simulink model "teste_motor_v10"  (R2025b)
settings: Solver=VariableStepAuto  StartTime=0.0  StopTime=10  RelTol=1e-3
undefined symbols (not defined in the file): fdesignblkfcn, gcbh, Kad, Kre
libraries: nesl_utility x26, fl_lib x25, simulink x19, dsparch4 x3, sdl_lib x2, simulink_extras x2, dspfdesign x1
(part 2 of 3)

== system teste_motor_v10/Motor de Sem Controle/Subsystem/Leituras/Janela ==
  In1 : Inport
  Aleatório : Subsystem
  Constant : Constant  Value=2
  Gain : Gain  Gain=1.5
  Janela : Subsystem
  Multiport Switch : MultiPortSwitch  SaturateOnIntegerOverflow=off  InputSameDT=off
  Product : Product
  Rotary Switch1 : CustomTuningWebBlock  LabelPosition=Hide  ShowInitialText=on  Configuration="{\"components\":[{\"name\":\"RotarySwitchComponent\",\"settings\":{\"arcAngle\":300,\"arcAngleOffset\":120,\"handle\":{\"size\":[150,150],\"src\":\"data:image\\/svg+xml;base64,PHN2ZyBpZD0iTGF5ZXJfMSIgZGF0YS1uYW1lPSJMYXllciAxIiB4bWxucz0iaHR0cDovL3d3dy53My5vcmcvMjAwMC9zdmciIHhtbG5zOnhsaW5rPSJodHRwOi8vd3d3LnczLm9yZy8xOTk5L3hsaW5rIiB2aWV3Qm94PSIwIDAgMTIxIDEyMSI+PGRlZnM+PHN0eWxlPi5jbHMtMXtmaWxsOnVybCgjbGluZWFyLWdyYWRpZW50KTt9LmNscy0yLC5jbHMtM3tmaWxsOiNkMWQxZDE7fS5jbHMtM3tzdHJva2U6I2I3YjdiNztzdHJva2UtbWl0ZXJsaW1pdDoxMDtzdHJva2Utd2lkdGg6MC4yNXB4O30uY2xzLTR7ZmlsbDojZjMwMDAwO30uY2xzLTV7ZmlsbDojZjIxNzY3O308L3N0eWxlPjxsaW5lYXJHcmFkaWVudCBpZD0ibGluZWFyLWdyYWRpZW50IiB4MT0iNjAuNSIgeTE9IjEyMC41IiB4Mj0iNjAuNSIgeTI9IjAuNSIgZ3JhZGllbnRVbml0cz0idXNlclNwYWNlT25Vc2UiPjxzdG9wIG9mZnNldD0iMCIgc3RvcC1jb2xvcj0iI2QxZDFkMSIvPjxzdG9wIG9mZnNldD0iMC4xIiBzdG9wLWNvbG9yPSIjY2VjZWNlIi8+PHN0b3Agb2Zmc2V0PSIwLjE5IiBzdG9wLWNvbG9yPSIjYzNjM2MzIi8+PHN0b3Agb2Zmc2V0PSIwLjI4IiBzdG9wLWNvbG9yPSIjYjFiMWIxIi8+PHN0b3Agb2Zmc2V0PSIwLjM2IiBzdG9wLWNvbG9yPSIjOTg5ODk4Ii8+PHN0b3Agb2Zmc2V0PSIwLjQ0IiBzdG9wLWNvbG9yPSIjNzg3ODc4Ii8+PHN0b3Agb2Zmc2V0PSIwLjQ2IiBzdG9wLWNvbG9yPSIjNmI2YjZiIi8+PHN0b3Agb2Zmc2V0PSIwLjU0IiBzdG9wLWNvbG9yPSIjNmI2YjZiIi8+PHN0b3Agb2Zmc2V0PSIwLjU2IiBzdG9wLWNvbG9yPSIjNzY3Njc2Ii8+PHN0b3Agb2Zmc2V0PSIwLjY0IiBzdG9wLWNvbG9yPSIjOTc5Nzk3Ii8+PHN0b3Agb2Zmc2V0PSIwLjcyIiBzdG9wLWNvbG9yPSIjYjBiMGIwIi8+PHN0b3Agb2Zmc2V0PSIwLjgxIiBzdG9wLWNvbG9yPSIjYzNjM2MzIi8+PHN0b3Agb2Zmc2V0PSIwLjkiIHN0b3AtY29sb3I9IiNjZGNkY2QiLz48c3RvcCBvZmZzZXQ9IjEiIHN0b3AtY29sb3I9IiNkMWQxZDEiLz48L2xpbmVhckdyYWRpZW50PjwvZGVmcz48Y2lyY2xlIGNsYXNzPSJjbHMtMSIgY3g9IjYwLjUiIGN5PSI2MC41IiByPSI2MCIvPjxwYXRoIGNsYXNzPSJjbHMtMiIgZD0iTTYwLjUsMUE1OS41LDU5LjUsMCwxLDEsMSw2MC41LDU5LjU3LDU5LjU3LDAsMCwxLDYwLjUsMW0wLTFBNjAuNSw2MC41LDAsMSwwLDEyMSw2MC41LDYwLjUsNjAuNSwwLDAsMCw2MC41LDBaIi8+PHJlY3QgY2xhc3M9ImNscy0zIiB4PSIwLjUiIHk9IjUxLjUiIHdpZHRoPSIxMjAiIGhlaWdodD0iMTgiIHJ4PSIzLjA0Ii8+PHJlY3QgY2xhc3M9ImNscy00IiB4PSI1Ljc1IiB5PSI1OC43NSIgd2lkdGg9IjE2IiBoZWlnaHQ9IjMiLz48cGF0aCBjbGFzcz0iY2xzLTUiIGQ9Ik0yMS4yNSw1OS4yNXYyaC0xNXYtMmgxNW0xLTFoLTE3djRoMTd2LTRaIi8+PC9zdmc+\"},\"handleOffset\":[0,0],\"handleOrientation\":180,\"handlePosition\":[0,0,1,1],\"handleSize\":{\"height\":0.5,\"width\":0.5},\"labelRadius\":0.36,\"position\":[0,0,1,1],\"states\":[{\"Label\":{\"color\":[0,0,0,1],\"icon\":{\"size\":[0,0],\"src\":[],\"srcOrientation\":\"Right\"},\"iconOffset\":0,\"iconPlacement\":\"left\",\"opacity\":1,\"position\":[0.35757211538461536,0.7603966346153846],\"show\":true,\"text\":{\"content\":\"Test\",\"font\":\"Helvetica\"}},\"Value\":1},{\"Label\":{\"color\":[0,0,0,1],\"icon\":{\"size\":[0,0],\"src\":[],\"srcOrientation\":\"Right\"},\"iconOffset\":0,\"iconPlacement\":\"left\",\"opacity\":1,\"position\":[0.09603365384615385,0.46033653846153844],\"show\":true,\"text\":{\"content\":\"Random\",\"font\":\"Helvetica\"}},\"Value\":2},{\"Label\":{\"color\":[0,0,0,1],\"icon\":{\"size\":[0,0],\"src\":[],\"srcOrientation\":\"Right\"},\"iconOffset\":0,\"iconPlacement\":\"left\",\"opacity\":1,\"position\":[0.36532451923076925,0.1180889423076923],\"show\":true,\"text\":{\"content\":\"Sequel\",\"font\":\"Helvetica\"}},\"Value\":3}],\"tickRadius\":0.32}},{\"name\":\"BackgroundImageComponent\",\"settings\":{\"image\":{\"size\":[155,150],\"src\":\"data:image\\/svg+xml;base64,PD94bWwgdmVyc2lvbj0iMS4wIiBlbmNvZGluZz0idXRmLTgiPz4NCjwhLS0gR2VuZXJhdG9yOiBBZG9iZSBJbGx1c3RyYXRvciAyNS4wLjAsIFNWRyBFeHBvcnQgUGx1Zy1JbiAuIFNWRyBWZXJzaW9uOiA2LjAwIEJ1aWxkIDApICAtLT4NCjxzdmcgdmVyc2lvbj0iMS4xIg0KCSBpZD0iTGF5ZXJfMl8xXyIgeG1sbnM6Y2M9Imh0dHA6Ly9jcmVhdGl2ZWNvbW1vbnMub3JnL25zIyIgeG1sbnM6ZGM9Imh0dHA6Ly9wdXJsLm9yZy9kYy9lbGVtZW50cy8xLjEvIiB4bWxuczppbmtzY2FwZT0iaHR0cDovL3d3dy5pbmtzY2FwZS5vcmcv ...(+4184 chars)\",\"srcOrientation\":\"Right\"},\"position\":[0,0,1,1],\"scaleMode\":\"0\"}},{\"name\":\"ForegroundImageComponent\",\"settings\":{\"image\":{\"size\":[0,0],\"src\":\"default\",\"srcOrientation\":[]},\"isForeground\":1,\"position\":[0,0,1,1],\"scaleMode\":\"0\"}}],\"derived\":{\"blockParameters\":{\"ForegroundColor\":[0.9882352941176471,0.9882352941176471,0.7725490196078432],\"SelectedStateIndex\":0,\"States\":[{\"Label\":{\"color\":[0,0,0,1],\"icon\":{\"size\":[0,0],\"src\":[],\"srcOrientation\":\"Right\"},\"iconOffset\":0,\"iconPlacement\":\"left\",\"opacity\":1,\"position\":[0.35757211538461536,0.7603966346153846],\"show\":true,\"text\":{\"content\":\"Test\",\"font\":\"Helvetica\"}},\"Value\":1},{\"Label\":{\"color\":[0,0,0,1],\"icon\":{\"size\":[0,0],\"src\":[],\"srcOrientation\":\"Right\"},\"iconOffset\":0,\"iconPlacement\":\"left\",\"opacity\":1,\"position\":[0.09603365384615385,0.46033653846153844],\"show\":true,\"text\":{\"content\":\"Random\",\"font\":\"Helvetica\"}},\"Value\":2},{\"Label\":{\"color\":[0,0,0,1],\"icon\":{\"size\":[0,0],\"src\":[],\"srcOrientation\":\"Right\"},\"iconOffset\":0,\"iconPlacement\":\"left\",\"opacity\":1,\"position\":[0.36532451923076925,0.1180889423076923],\"show\":true,\"text\":{\"content\":\"Sequel\",\"font\":\"Helvetica\"}},\"Value\":3}],\"StatesJSON\":[{\"Label\":\"Test\",\"Value\":1},{\"Label\":\"Random\",\"Value\":2},{\"Label\":\"Sequel\",\"Value\":3}],\"enumDataType\":\"\",\"fixedAspectRatio\":\"on\",\"useEnumDataType\":false}},\"settings\":{\"BindingType\":\"param\",\"backgroundColor\":[0,0,255,\"1\"],\"backgroundOffset\":1,\"fixedAspectRatio\":\"on\",\"image\":{\"size\":[150,150],\"src\":\"data:image\\/svg+xml;base64,PD94bWwgdmVyc2lvbj0iMS4wIiBlbmNvZGluZz0iVVRGLTgiIHN0YW5kYWxvbmU9Im5vIj8+CjwhLS0gR2VuZXJhdG9yOiBBZG9iZSBJbGx1c3RyYXRvciAxOS4yLjEsIFNWRyBFeHBvcnQgUGx1Zy1JbiAuIFNWRyBWZXJzaW9uOiA2LjAwIEJ1aWxkIDApICAtLT4KCjxzdmcKICAgeG1sbnM6ZGM9Imh0dHA6Ly9wdXJsLm9yZy9kYy9lbGVtZW50cy8xLjEvIgogICB4bWxuczpjYz0iaHR0cDovL2NyZWF0aXZlY29tbW9ucy5vcmcvbnMjIgogICB4bWxuczpyZGY9Imh0dHA6Ly93d3cudzMub3JnLzE5OTkvMDIvMjItcmRmLXN5bnRh ...(+9660 chars)\"},\"showBackgroundColor\":false,\"variant\":\"rotarySwitch\",\"version\":\"R2023a\"},\"type\":\"RotarySwitch\"}"
  Sequência : Subsystem
  Teste : Subsystem
  Out1 : Outport
  wires:
  In1/1 -> Janela/1(In1)
  Janela/1(Output) -> Product/2
  Product/1 -> Gain/1
  Gain/1 -> Out1/1
  Constant/1 -> Multiport Switch/1
  Teste/1(Out1) -> Multiport Switch/2
  Sequência/1(3) -> Multiport Switch/4
  Aleatório/1(2) -> Multiport Switch/3
  Multiport Switch/1 -> Product/1

== system teste_motor_v10/Motor de Sem Controle/Subsystem/Leituras/Knock ==
  In1 : Inport
  Abs1 : Abs  SaturateOnIntegerOverflow=off
  MATLAB Function : MATLAB Function  TreatAsAtomicUnit=on
  Product : Product  Inputs=3
  Transfer Fcn : TransferFcn  Denominator=[0.0002 1]
  Uniform Random Number : UniformRandomNumber  Minimum=1800  Maximum=2000  SampleTime=0.0001
  Waveform Generator : simulink/Sources/Waveform Generator  OutMin=[]  OutMax=[]  OutDataTypeStr=double  SelectedSignal=1  Signals=sin(1,80000,1)  BlockNames=MultiportSwitch_adaf1d14f166474  SampleTime=0.1
  Out1 : Outport
  wires:
  Waveform Generator/1 -> Abs1/1
  Transfer Fcn/1 -> Product/3
  Abs1/1 -> Product/2
  Product/1 -> Out1/1
  In1/1 -> Transfer Fcn/1
  MATLAB Function/1(knock_probabilidade) -> Product/1
  [rpm] -> MATLAB Function/1(rpm)
  [AFR] -> MATLAB Function/2(AFR)
  [sa] -> MATLAB Function/3(SA)

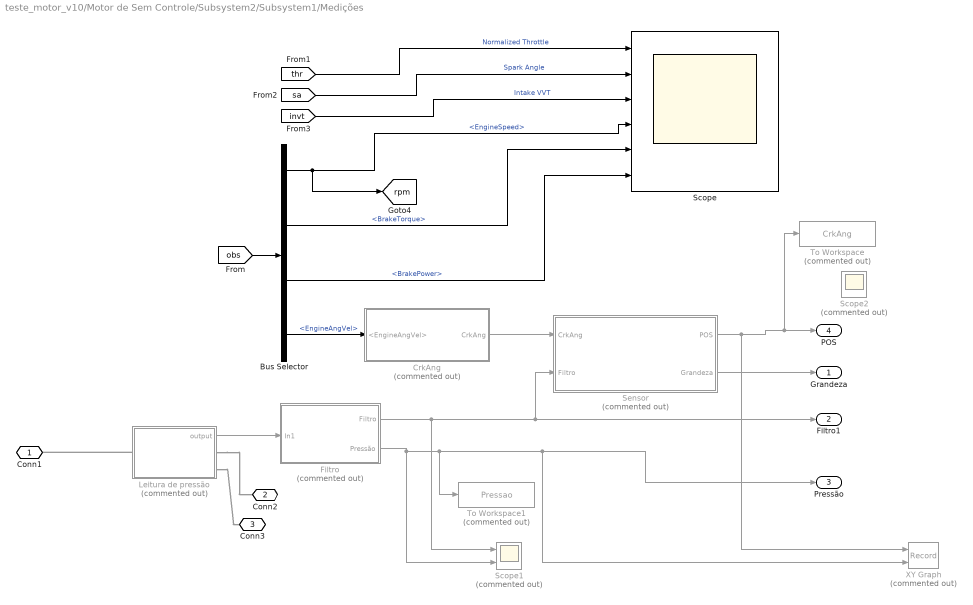
== system teste_motor_v10/Motor de Sem Controle/Subsystem2/Subsystem1/Medições ==
  Bus Selector : BusSelector  OutputSignals=EngineSpeed,BrakeTorque,BrakePower,EngineAngVel
  CrkAng : Subsystem  Commented=on
  Filtro : Subsystem  Commented=on
  Leitura de pressão : Subsystem  Commented=on
  Scope : Scope  NumInputPorts=6
      settings: ActiveDisplayYMinimum=0.1  ActiveDisplayYMaximum=1.1
  Scope1 : Scope  Commented=on  NumInputPorts=2
      settings: ActiveDisplayYMinimum=-2759.66095  ActiveDisplayYMaximum=3628.39198  DataLoggingVariableName=ScopeData3
  Scope2 : Scope  Commented=on
      settings: ActiveDisplayYMinimum=-46.25  ActiveDisplayYMaximum=416.25
  Sensor : Subsystem  Commented=on
  To Workspace : ToWorkspace  Commented=on  VariableName=CrkAng  SaveFormat=Timeseries  SampleTime=-1
  To Workspace1 : ToWorkspace  Commented=on  VariableName=Pressao  SaveFormat=Timeseries  SampleTime=-1
  XY Graph : Record  Commented=on  NumPorts=2.0  FileSettingsInternal="{\"entries\":[{\"content\":{\"excelSettings\":{\"content\":{},\"type\":\"Streamout.ExcelSettings\"},\"parquetSettings\":{\"content\":{},\"type\":\"Streamout.ParquetSettings\"}},\"type\":\"Streamout.FileSettingStorage\",\"uuid\":\"\"}],\"packageUris\":[\"http:\\/\\/schema.mathworks.com\\/mf0\\/streamout_blocks\\/R2020a\"],\"version\":\"1.0\"}"  FrameSettings=[0, 0]  Layout=[1 1]  SignalsInternal="{\"entries\":[{\"content\":{},\"type\":\"RecordBlkView.InputSignals\",\"uuid\":\"\"}],\"packageUris\":[\"http:\\/\\/schema.mathworks.com\\/mf0\\/streamout_blocks\\/R2020a\"],\"version\":\"1.0\"}"  VisualizationBindings="{\"xyplotplugin\":{\"info\":[{\"series\":[],\"subplotID\":1}]}}"  CompatibilityTag=XY
  Conn1 : PMIOPort  Side=Left
  Conn2 : PMIOPort  Port=2  Side=Right
  Conn3 : PMIOPort  Port=3  Side=Right
  Grandeza : Outport
  Filtro1 : Outport  Port=2
  Pressão : Outport  Port=3
  POS : Outport  Port=4
  tag scope: rpm=global
  wires:
  [invt] -> Scope/3  "Intake VVT"
  CrkAng/1(CrkAng) -> Sensor/1(CrkAng)
  Filtro/1(Filtro) -> Scope1/1, Filtro1/1, Sensor/2(Filtro)
  [obs] -> Bus Selector/1
  Bus Selector/4 -> CrkAng/1(<EngineAngVel>)  "<EngineAngVel>"
  Leitura de pressão/1(output) -> Filtro/1(In1)
  Bus Selector/2 -> Scope/5  "<BrakeTorque>"
  Bus Selector/3 -> Scope/6  "<BrakePower>"
  Bus Selector/1 -> [rpm], Scope/4  "<EngineSpeed>"
  [sa] -> Scope/2  "Spark Angle"
  [thr] -> Scope/1  "Normalized Throttle"
  Sensor/2(Grandeza) -> Grandeza/1
  Sensor/1(POS) -> XY Graph/1, To Workspace/1, POS/1
  Filtro/2(Pressão) -> Scope1/2, To Workspace1/1, XY Graph/2, Pressão/1
  connections:
  Leitura de pressão/RConn1 -- Conn2/RConn1
  Leitura de pressão/LConn1 -- Conn1/RConn1
  Leitura de pressão/RConn2 -- Conn3/RConn1

== system teste_motor_v10/Motor de com Controle/Medições/Filtro/Bandpass Filter ==
  In : Inport
  Generated Filter Block : dsparch4/Biquad Filter  Tag=BlockMethodSubSystem  FilterSource=Dialog parameters  CoeffSource=Specify via dialog  FilterObject=BQF  IIRFiltStruct=Direct form II  BiQuadCoeffs=[2 0 -2 1 1.83695911000028955 0.883333019360894145]  ScaleValues=[0.0247421229251508536;1.1788295308373844]  IC=0  ICnum=0  ICden=0  a0Flag=Warning  optimizeScaleValues=off  ScaleValueMode=Specify via input port (g)  InputProcessing=Columns as channels (frame based)  roundingMode=Floor  overflowMode=off  scaleValueFracLength=14  denProdOutputFracLength=30  denAccumFracLength=30  secondMemoryFracLength=15
  Out : Outport  VectorParamsAs1DForOutWhenUnconnected=off
  wires:
  In/1 -> Generated Filter Block/1
  Generated Filter Block/1 -> Out/1

== system teste_motor_v10/Motor de com Controle/Medições/Filtro/Subsystem1 ==
  RPM : Inport
  Constant1 : Constant  Value=15
  Constant2 : Constant  Value=0
  Display : Display
  Product1 : Product
  Scope : Scope
      settings: ActiveDisplayYMinimum=-37.46596  ActiveDisplayYMaximum=337.1936
  Scope1 : Scope
      settings: ActiveDisplayYMinimum=-0.125  ActiveDisplayYMaximum=1.125
  Step : Step  Time=45  Before=15  After=20  SampleTime=0
  Subsystem : Subsystem
  Sum1 : Sum
  Uniform Random Number : UniformRandomNumber  Minimum=0  Maximum=300  SampleTime=0.1
  Output : Outport
  wires:
  Sum1/1 -> Output/1, Display/1, Scope/1
  Subsystem/1(knock) -> Scope1/1, Product1/1
  Constant1/1 -> Subsystem/1(Rel Spark)
  RPM/1 -> Subsystem/2(RPM)
  Product1/1 -> Sum1/1
  Constant2/1 -> Sum1/2
  Uniform Random Number/1 -> Product1/2

== system teste_motor_v10/Motor de com Controle/Medições/Filtro/Subsystem2 ==
  RPM : Inport
  Constant1 : Constant  Value=15
  Data Type Conversion : DataTypeConversion  OutDataTypeStr=double  SaturateOnIntegerOverflow=off  RndMeth=Floor
  Data Type Conversion1 : DataTypeConversion  OutDataTypeStr=double  SaturateOnIntegerOverflow=off  RndMeth=Floor
  Data Type Conversion2 : DataTypeConversion  OutDataTypeStr=boolean  SaturateOnIntegerOverflow=off  RndMeth=Floor
  Display : Display
  Product1 : Product
  S-R Flip-Flop : simulink_extras/Flip Flops/S-R Flip-Flop  initial_condition=0
  Scope : Scope
      settings: ActiveDisplayYMinimum=-37.46596  ActiveDisplayYMaximum=337.1936
  Scope1 : Scope
      settings: ActiveDisplayYMinimum=-0.125  ActiveDisplayYMaximum=1.125
  Subsystem : Subsystem
  Transport Delay : TransportDelay  DelayTime=9.9
  Uniform Random Number : UniformRandomNumber  Minimum=1000  Maximum=2000  SampleTime=10
  Output : Outport
  wires:
  Product1/1 -> Output/1, Display/1, Scope/1
  Constant1/1 -> Subsystem/1(Rel Spark)
  RPM/1 -> Subsystem/2(RPM)
  Uniform Random Number/1 -> Product1/2
  Subsystem/1(knock) -> Data Type Conversion1/1, S-R Flip-Flop/1
  S-R Flip-Flop/1 -> Scope1/1, Data Type Conversion/1
  Data Type Conversion/1 -> Product1/1
  Data Type Conversion1/1 -> Transport Delay/1
  Data Type Conversion2/1 -> S-R Flip-Flop/2
  Transport Delay/1 -> Data Type Conversion2/1

== system teste_motor_v10/Motor de com Controle/Medições/Sensor/Sensor ==
  In1 : Inport
  In2 : Inport  Port=2
  Constant : Constant  Value=720
  Constant1 : Constant  Value=370
  Constant2 : Constant  Value=410
  Detect Rise Positive : simulink/Logic and Bit Operations/Detect Rise Positive  vinit=0  OutDataTypeStr=boolean
  Leitura do sensor : Math  Operator=square
  Logical Operator : Logic  AllPortsSameDT=off  OutDataTypeStr=boolean
  Mod : Math  Operator=mod
  Product : Product
  Relational Operator : RelationalOperator  OutDataTypeStr=boolean  RndMeth=Simplest  InputSameDT=off
  Relational Operator1 : RelationalOperator  Operator=<=  OutDataTypeStr=boolean  RndMeth=Simplest  InputSameDT=off
  Threshold : simulink/Logic and Bit Operations/Compare To Constant  relop=>  const=1  OutDataTypeStr=boolean
  Output : Outport
  wires:
  Relational Operator1/1 -> Logical Operator/2
  Relational Operator/1 -> Logical Operator/1
  Constant1/1 -> Relational Operator/1
  Mod/1 -> Relational Operator1/1, Relational Operator/2
  Constant2/1 -> Relational Operator1/2
  Logical Operator/1 -> Product/1
  Detect Rise Positive/1 -> Output/1
  Constant/1 -> Mod/2
  Leitura do sensor/1 -> Threshold/1
  Product/1 -> Leitura do sensor/1
  Threshold/1 -> Detect Rise Positive/1
  In1/1 -> Mod/1
  In2/1 -> Product/2

== system teste_motor_v10/Motor de com Controle/Medições/Sensor/Subsystem4 ==
  u : Inport
  Subsystem : Subsystem
  Subsystem1 : Subsystem
  Subsystem3 : Subsystem
  Out1 : Outport
  wires:
  u/1 -> Subsystem3/1(In1), Subsystem1/1(u), Subsystem/1(u)
  Subsystem1/1(Contagem) -> Subsystem3/2(u)
  Subsystem3/1(Out1) -> Out1/1
  Subsystem/1(Borda de Subida) -> Subsystem3/3(In3)

== system teste_motor_v10/Motor de Sem Controle/Subsystem/Leituras/Janela/Aleatório ==
  Compare To Constant : simulink/Logic and Bit Operations/Compare To Constant  relop=>  const=0.99  OutDataTypeStr=boolean
  Uniform Random Number : UniformRandomNumber  SampleTime=0.0001
  2 : Outport
  wires:
  Uniform Random Number/1 -> Compare To Constant/1
  Compare To Constant/1 -> 2/1

== system teste_motor_v10/Motor de Sem Controle/Subsystem/Leituras/Janela/Janela ==
  In1 : Inport
  Constant2 : Constant  Value=385
  Constant3 : Constant  Value=390
  Data Type Conversion : DataTypeConversion  OutDataTypeStr=double  SaturateOnIntegerOverflow=off  RndMeth=Floor
  Logical Operator : Logic  AllPortsSameDT=off  OutDataTypeStr=boolean
  Relational Operator : RelationalOperator  Operator=<=  OutDataTypeStr=boolean  RndMeth=Simplest  InputSameDT=off
  Relational Operator1 : RelationalOperator  Operator=<=  OutDataTypeStr=boolean  RndMeth=Simplest  InputSameDT=off
  Scope : Scope  NumInputPorts=2
      settings: ActiveDisplayYMinimum=-75.66542  ActiveDisplayYMaximum=430.14574  DataLoggingVariableName=ScopeData5
  Output : Outport
  wires:
  Relational Operator/1 -> Logical Operator/1
  Constant2/1 -> Relational Operator/1
  Logical Operator/1 -> Scope/1, Data Type Conversion/1
  In1/1 -> Scope/2, Relational Operator1/1, Relational Operator/2
  Constant3/1 -> Relational Operator1/2
  Relational Operator1/1 -> Logical Operator/2
  Data Type Conversion/1 -> Output/1

== system teste_motor_v10/Motor de Sem Controle/Subsystem/Leituras/Janela/Sequência ==
  Step2 : Step  Time=0.2  SampleTime=0
  3 : Outport
  wires:
  Step2/1 -> 3/1

== system teste_motor_v10/Motor de Sem Controle/Subsystem/Leituras/Janela/Teste ==
  Step : Step  Time=0.5  SampleTime=0
  Step1 : Step  Time=0.7  SampleTime=0
  Subtract : Sum  Inputs=+-
  Out1 : Outport
  wires:
  Step1/1 -> Subtract/2
  Step/1 -> Subtract/1
  Subtract/1 -> Out1/1

== system teste_motor_v10/Motor de Sem Controle/Subsystem2/Subsystem1/Medições/CrkAng ==
  <EngineAngVel> : Inport
  Constant : Constant  Value=720
  Gain : Gain  Gain=180/pi
  Integrator : Integrator
  Mod : Math  Operator=mod
  CrkAng : Outport
  wires:
  Gain/1 -> Mod/1
  Integrator/1 -> Gain/1
  <EngineAngVel>/1 -> Integrator/1
  Mod/1 -> CrkAng/1
  Constant/1 -> Mod/2

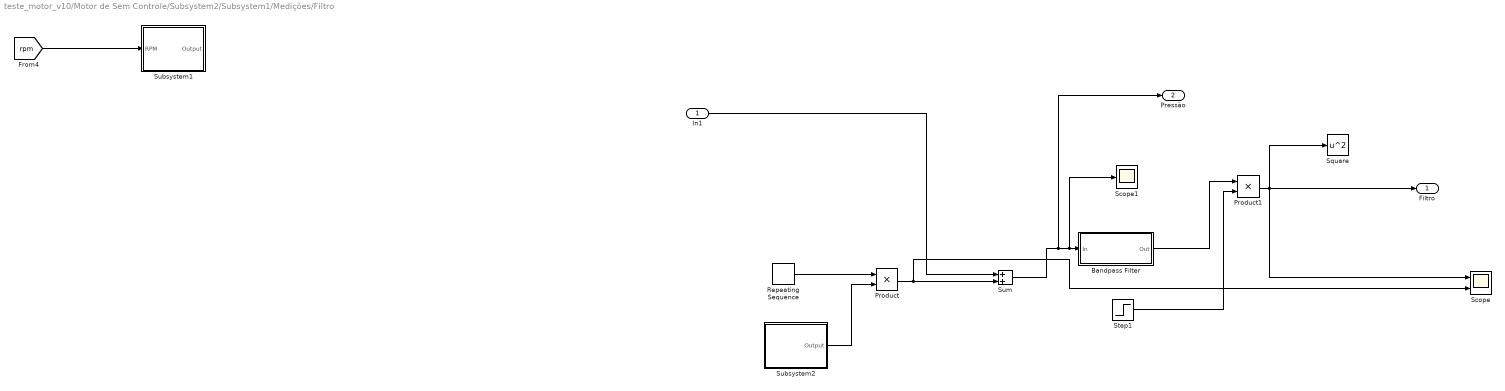
== system teste_motor_v10/Motor de Sem Controle/Subsystem2/Subsystem1/Medições/Filtro ==
  In1 : Inport
  Bandpass Filter : Subsystem  DialogController=fdesignblkfcn  InitFcn=fdesignblkfcn(gcbh, {'InitFcn'});  mask(Bandpass Filter){}
      mask help: Design a bandpass filter
      settings: CopyFcn=fdesignblkfcn(gcbh, {'CopyFcn'});
      mask Help: helpview(mapfilelocation('dsp'), 'dspbandpassfilter');
      mask Display: disp('Bandpass');
  Product : Product
  Product1 : Product
  Repeating Sequence : simulink/Sources/Repeating Sequence  rep_seq_t=[0, 1]  rep_seq_y=[1, 1]
  Scope : Scope  NumInputPorts=2
      settings: ActiveDisplayYMinimum=-2759.66095  ActiveDisplayYMaximum=3628.39198  DataLoggingVariableName=ScopeData2
  Scope1 : Scope
      settings: ActiveDisplayYMinimum=101167.74999  ActiveDisplayYMaximum=102740.25008  DataLoggingVariableName=ScopeData8
  Square : Math  Operator=square
  Step1 : Step  Time=10  SampleTime=0
  Subsystem1 : Subsystem
  Subsystem2 : Subsystem
  Sum : Sum
  Filtro : Outport
  Pressão : Outport  Port=2
  wires:
  Bandpass Filter/1(Out) -> Product1/1
  [rpm] -> Subsystem1/1(RPM)
  Product1/1 -> Filtro/1, Square/1, Scope/1
  In1/1 -> Sum/1
  Subsystem2/1(Output) -> Product/2
  Repeating Sequence/1 -> Product/1
  Product/1 -> Scope/2, Sum/2
  Step1/1 -> Product1/2
  Sum/1 -> Pressão/1, Scope1/1, Bandpass Filter/1(In)

== system teste_motor_v10/Motor de Sem Controle/Subsystem2/Subsystem1/Medições/Leitura de pressão ==
  Absolute Reference (G) : fl_lib/Gas/Elements/Absolute Reference (G)
      settings: InternalSimscapePortConfiguration="{\"Bottom\":[],\"Left\":[{\"id\":\"A\",\"label\":\"\",\"type\":\"foundation.gas.gas\"}],\"Right\":[],\"Top\":[]}"
  Engine Friction : fl_lib/Mechanical/Rotational Elements/Rotational Damper  D=0.01 N*m/rpm  w_specify=off  w_priority=None  w=0 rad/s  w_nominal_specify=off  w_nominal_value=1  w_nominal_unit=rad/s  t_specify=off  t_priority=None  t=0 N*m  t_nominal_specify=off  t_nominal_value=1  t_nominal_unit=N*m
      settings: AttributesFormatString=%<D> [%<D_unit>]
  Mechanical Rotational Reference1 : fl_lib/Mechanical/Rotational Elements/Mechanical Rotational Reference
  PS-Simulink Converter4 : nesl_utility/PS-Simulink Converter  PhysicalDomain=network_engine_domain  SubClassName=ps_output  LeftPortType=input  RightPortType=output  PseudoPeriodic=off  Frequencies=[]  VectorFormat=inherit  Unit=Pa  AffineConversion=off
  Pressure & Temperature Sensor (G) : fl_lib/Gas/Sensors/Pressure & Temperature Sensor (G)  reference=foundation.enum.MeasurementReference.difference  pressure=true  pressure_spec=foundation.enum.PressureMeasementSpec.Absolute  temperature=true
      settings: InternalSimscapePortConfiguration="{\"Bottom\":[{\"id\":\"T\",\"label\":\"T\",\"type\":\"output\"}],\"Left\":[{\"id\":\"A\",\"label\":\"A\",\"type\":\"foundation.gas.gas\"}],\"Right\":[{\"id\":\"B\",\"label\":\"B\",\"type\":\"foundation.gas.gas\"},{\"id\":\"P\",\"label\":\"P\",\"type\":\"output\"}],\"Top\":[]}"
  Rotational Mechanical Converter (G) : fl_lib/Gas/Elements/Rotational Mechanical Converter (G)  mech_orientation=foundation.enum.MechOrientationRotational.Negative  rotation_spec=foundation.enum.RotationSpec.Calculate  theta_init=0 rad  volume_displacement=0.01 m^3/rad  dead_volume=1e-5 m^3  area_A=0.01 m^2  environment_spec=foundation.enum.pressure_spec.atmospheric  environment_pressure=0.101325 MPa  p_I_specify=off  p_I_priority=High  p_I=0.101325 MPa  p_I_nominal_specify=off  p_I_nominal_value=1  p_I_nominal_unit=MPa  T_I_specify=off  T_I_priority=High  T_I=293.15 K  T_I_nominal_specify=off  T_I_nominal_value=1  T_I_nominal_unit=K  rho_I_specify=off  rho_I_priority=High  rho_I=0.715 kg/m^3  rho_I_nominal_specify=off  rho_I_nominal_value=1  rho_I_nominal_unit=kg/m^3
      settings: InternalSimscapePortConfiguration="{\"Bottom\":[],\"Left\":[{\"id\":\"A\",\"label\":\"A\",\"type\":\"foundation.gas.gas\"},{\"id\":\"R\",\"label\":\"R\",\"type\":\"foundation.mechanical.rotational.rotational\"}],\"Right\":[{\"id\":\"H\",\"label\":\"H\",\"type\":\"foundation.thermal.thermal\"},{\"id\":\"C\",\"label\":\"C\",\"type\":\"foundation.mechanical.rotational.rotational\"}],\"Top\":[]}"
  Conn1 : PMIOPort  Side=Left
  Conn2 : PMIOPort  Port=2  Side=Right
  Conn3 : PMIOPort  Port=3  Side=Right
  output : Outport
  wires:
  PS-Simulink Converter4/1 -> output/1
  connections:
  Pressure & Temperature Sensor (G)/RConn3 -- Conn2/RConn1
  Rotational Mechanical Converter (G)/LConn1 -- Pressure & Temperature Sensor (G)/LConn1
  Pressure & Temperature Sensor (G)/RConn2 -- PS-Simulink Converter4/LConn1
  Rotational Mechanical Converter (G)/RConn1 -- Conn3/RConn1
  Pressure & Temperature Sensor (G)/RConn1 -- Absolute Reference (G)/LConn1
  Rotational Mechanical Converter (G)/LConn2 -- Conn1/RConn1
  Mechanical Rotational Reference1/LConn1 -- Engine Friction/RConn1
  Engine Friction/LConn1 -- Rotational Mechanical Converter (G)/RConn2

== system teste_motor_v10/Motor de Sem Controle/Subsystem2/Subsystem1/Medições/Sensor ==
  CrkAng : Inport
  Filtro : Inport  Port=2
  Product : Product
  Scope : Scope
      settings: ActiveDisplayYMinimum=-1  ActiveDisplayYMaximum=1  DataLoggingVariableName=ScopeData7
  Sensor : Subsystem
  Square : Math  Operator=square
  Square Root : Sqrt
  Subsystem4 : Subsystem
  POS : Outport
  Grandeza : Outport  Port=2
  wires:
  CrkAng/1 -> Sensor/1(In1)
  Filtro/1 -> Sensor/2(Sinal do filtro), Product/2
  Square Root/1 -> Grandeza/1
  Product/1 -> Square/1
  Square/1 -> Square Root/1
  Subsystem4/1(Out1) -> Scope/1, Product/1
  Sensor/2(Output) -> Subsystem4/1(u)
  Sensor/1(POS) -> POS/1

== system teste_motor_v10/Motor de com Controle/Medições/Filtro/Subsystem1/Subsystem ==
  Rel Spark : Inport
  RPM : Inport  Port=2
  2-D Lookup Table : Lookup_n-D  BreakpointsForDimension1=[12, 17, 20, 25, 30]  BreakpointsForDimension2=[200, 400, 800, 1000, 2000]  Table=[0 0 0 0 0; 0.05 0.05 0.02 0.01 0.01; 0.2 0.15 0.1 0.05 0.05; 0.6 0.5 0.3 0.2 0.1; 0.95 0.9 0.8 0.6 0.4]  InternalRulePriority=Speed  RndMeth=Simplest
      settings: InputPortMap=u0,u1
  Constant4 : Constant
  Relational Operator : RelationalOperator  Operator=<  OutDataTypeStr=boolean  RndMeth=Simplest  InputSameDT=off
  Subtract : Sum  Inputs=+-
  Uniform Random Number : UniformRandomNumber  Minimum=0  SampleTime=0.1
  Unit Delay : UnitDelay  SampleTime=-1  HasFrameUpgradeWarning=on
  knock : Outport
  wires:
  2-D Lookup Table/1 -> Subtract/2
  RPM/1 -> 2-D Lookup Table/2
  Relational Operator/1 -> Unit Delay/1
  Unit Delay/1 -> knock/1
  Rel Spark/1 -> 2-D Lookup Table/1
  Uniform Random Number/1 -> Relational Operator/2
  Subtract/1 -> Relational Operator/1
  Constant4/1 -> Subtract/1

== system teste_motor_v10/Motor de com Controle/Medições/Filtro/Subsystem2/Subsystem ==
  Rel Spark : Inport
  RPM : Inport  Port=2
  2-D Lookup Table : Lookup_n-D  BreakpointsForDimension1=[12, 17, 20, 25, 30]  BreakpointsForDimension2=[200, 400, 800, 1000, 2000]  Table=[0 0 0 0 0; 0.05 0.05 0.02 0.01 0.01; 0.2 0.15 0.1 0.05 0.05; 0.6 0.5 0.3 0.2 0.1; 0.95 0.9 0.8 0.6 0.4]  InternalRulePriority=Speed  RndMeth=Simplest
      settings: InputPortMap=u0,u1
  Constant4 : Constant
  Relational Operator : RelationalOperator  Operator=<  OutDataTypeStr=boolean  RndMeth=Simplest  InputSameDT=off
  Subtract : Sum  Inputs=+-
  Uniform Random Number : UniformRandomNumber  Minimum=0  SampleTime=0.1
  Unit Delay : UnitDelay  SampleTime=-1  HasFrameUpgradeWarning=on
  knock : Outport
  wires:
  2-D Lookup Table/1 -> Subtract/2
  RPM/1 -> 2-D Lookup Table/2
  Relational Operator/1 -> Unit Delay/1
  Unit Delay/1 -> knock/1
  Rel Spark/1 -> 2-D Lookup Table/1
  Uniform Random Number/1 -> Relational Operator/2
  Subtract/1 -> Relational Operator/1
  Constant4/1 -> Subtract/1

== system teste_motor_v10/Motor de com Controle/Medições/Sensor/Subsystem4/Subsystem ==
  u : Inport
  AND : Logic  Inputs=3  IconShape=distinctive  AllPortsSameDT=off  OutDataTypeStr=boolean
  Compare To Constant : simulink/Logic and Bit Operations/Compare To Constant  relop=>  const=0  OutDataTypeStr=boolean
  Compare To Constant1 : simulink/Logic and Bit Operations/Compare To Constant  relop=>  const=0  OutDataTypeStr=boolean
  NOT : Logic  Operator=NOT  IconShape=distinctive  AllPortsSameDT=off  OutDataTypeStr=boolean
  Unit Delay : UnitDelay  SampleTime=-1  HasFrameUpgradeWarning=on
  Borda de Subida : Outport
  wires:
  u/1 -> Compare To Constant1/1, AND/2, Compare To Constant/1
  Unit Delay/1 -> NOT/1
  AND/1 -> Borda de Subida/1
  NOT/1 -> AND/1
  Compare To Constant/1 -> Unit Delay/1
  Compare To Constant1/1 -> AND/3

== system teste_motor_v10/Motor de com Controle/Medições/Sensor/Subsystem4/Subsystem1 ==
  u : Inport
  Compare To Constant : simulink/Logic and Bit Operations/Compare To Constant  relop===  const=0  OutDataTypeStr=boolean
  Constant : Constant
  Constant1 : Constant  Value=0
  Sum : Sum
  Switch : Switch  Criteria=u2 > Threshold  SaturateOnIntegerOverflow=off  InputSameDT=off
  Unit Delay : UnitDelay  SampleTime=-1  HasFrameUpgradeWarning=on
  Contagem : Outport
  wires:
  Compare To Constant/1 -> Switch/2
  Unit Delay/1 -> Contagem/1, Sum/1
  Constant1/1 -> Switch/3
  Sum/1 -> Switch/1
  Switch/1 -> Unit Delay/1
  u/1 -> Compare To Constant/1
  Constant/1 -> Sum/2

== system teste_motor_v10/Motor de com Controle/Medições/Sensor/Subsystem4/Subsystem3 ==
  In1 : Inport
  u : Inport  Port=2
  In3 : Inport  Port=3
  AND : Logic  IconShape=distinctive  AllPortsSameDT=off  OutDataTypeStr=boolean
  Compare To Constant : simulink/Logic and Bit Operations/Compare To Constant  relop=>=  const=10  OutDataTypeStr=boolean
  Constant : Constant  Value=0
  Switch : Switch  Criteria=u2 > Threshold  SaturateOnIntegerOverflow=off  InputSameDT=off
  Out1 : Outport
  wires:
  u/1 -> Compare To Constant/1
  In1/1 -> Switch/1
  AND/1 -> Switch/2
  Compare To Constant/1 -> AND/1
  Constant/1 -> Switch/3
  Switch/1 -> Out1/1
  In3/1 -> AND/2

== system teste_motor_v10/Motor de Sem Controle/Subsystem2/Subsystem1/Medições/Filtro/Bandpass Filter ==
  In : Inport
  Generated Filter Block : dsparch4/Biquad Filter  Tag=BlockMethodSubSystem  FilterSource=Dialog parameters  CoeffSource=Specify via dialog  FilterObject=BQF  IIRFiltStruct=Direct form II  BiQuadCoeffs=[0.140685454860889653 0 -0.140685454860889653 1 -1.85912341066970588 0.867737263035942452;0.346083312765764206 0 -0.346083312765764206 1 -1.78434455590640884 0.797889421035578805;0.397474560674797361 0 -0.397474560674797361 1 -1.55910049254939209 0.6146704037687728;0.0137782157172320115 0 -0.0137782157172320115 1 -1.51950945901080425 0.60912544450482442;0.0250316410593518085 0 -0.0250316410593518085 1 -1.97790364921706252 0.983498174477606124;0.927629619481280199 0 -0.927629619481280199 1 -1.94406459171441304 0.94997302880633927;0.750019431315798291 0 -0.750019431315798291 1 -1.6190153742305462 0.766745360322838576;0.0436738551579278697 0 -0.0436738551579278697 1 -1.54442120528411775 0.664455129285150492;1.02538053332798063 0 -1.02538053332798063 1 -1.90636519119939529 0.913125075301058131;2 0 -2 1 -1.7410555566743704 0.912319021633544835]  ScaleValues=[0.00861385236623646126;1;1;1;1;1;1;1;1;1;2.95431131952925385]  IC=0  ICnum=0  ICden=0  a0Flag=Warning  optimizeScaleValues=off  ScaleValueMode=Specify via input port (g)  InputProcessing=Columns as channels (frame based)  roundingMode=Floor  overflowMode=off  scaleValueFracLength=14  denProdOutputFracLength=30  denAccumFracLength=30  secondMemoryFracLength=15
  Out : Outport  VectorParamsAs1DForOutWhenUnconnected=off
  wires:
  In/1 -> Generated Filter Block/1
  Generated Filter Block/1 -> Out/1

== system teste_motor_v10/Motor de Sem Controle/Subsystem2/Subsystem1/Medições/Filtro/Subsystem1 ==
  RPM : Inport
  Constant1 : Constant  Value=15
  Constant2 : Constant  Value=0
  Display : Display
  Product1 : Product
  Scope : Scope
      settings: ActiveDisplayYMinimum=-37.46596  ActiveDisplayYMaximum=337.1936
  Scope1 : Scope
      settings: ActiveDisplayYMinimum=-0.125  ActiveDisplayYMaximum=1.125
  Step : Step  Time=45  Before=15  After=20  SampleTime=0
  Subsystem : Subsystem
  Sum1 : Sum
  Uniform Random Number : UniformRandomNumber  Minimum=0  Maximum=300  SampleTime=0.1
  Output : Outport
  wires:
  Sum1/1 -> Output/1, Display/1, Scope/1
  Subsystem/1(knock) -> Scope1/1, Product1/1
  Constant1/1 -> Subsystem/1(Rel Spark)
  RPM/1 -> Subsystem/2(RPM)
  Product1/1 -> Sum1/1
  Constant2/1 -> Sum1/2
  Uniform Random Number/1 -> Product1/2

== system teste_motor_v10/Motor de Sem Controle/Subsystem2/Subsystem1/Medições/Filtro/Subsystem2 ==
  Constant1 : Constant  Commented=on  Value=15
  Data Type Conversion : DataTypeConversion  Commented=on  OutDataTypeStr=double  SaturateOnIntegerOverflow=off  RndMeth=Floor
  Data Type Conversion1 : DataTypeConversion  Commented=on  OutDataTypeStr=double  SaturateOnIntegerOverflow=off  RndMeth=Floor
  Data Type Conversion2 : DataTypeConversion  Commented=on  OutDataTypeStr=boolean  SaturateOnIntegerOverflow=off  RndMeth=Floor
  Display : Display
  Product1 : Product
  Pulse Generator : DiscretePulseGenerator  Period=5000  PulseWidth=1000  PhaseDelay=3000  SampleTime=0.01
  S-R Flip-Flop : simulink_extras/Flip Flops/S-R Flip-Flop  Commented=on  initial_condition=0
  Scope : Scope
      settings: ActiveDisplayYMinimum=-29.48241  ActiveDisplayYMaximum=265.34169
  Scope1 : Scope  Commented=on
      settings: ActiveDisplayYMinimum=-0.125  ActiveDisplayYMaximum=1.125
  Subsystem : Subsystem  Commented=on
  Transport Delay : TransportDelay  Commented=on  DelayTime=0.1
  Uniform Random Number : UniformRandomNumber  Minimum=150  Maximum=300  SampleTime=10
  Output : Outport
  wires:
  Product1/1 -> Output/1, Display/1, Scope/1
  Constant1/1 -> Subsystem/1(Rel Spark)
  Uniform Random Number/1 -> Product1/2
  Subsystem/1(knock) -> Data Type Conversion1/1, S-R Flip-Flop/1
  S-R Flip-Flop/1 -> Scope1/1, Data Type Conversion/1
  Data Type Conversion1/1 -> Transport Delay/1
  Data Type Conversion2/1 -> S-R Flip-Flop/2
  Transport Delay/1 -> Data Type Conversion2/1
  Pulse Generator/1 -> Product1/1

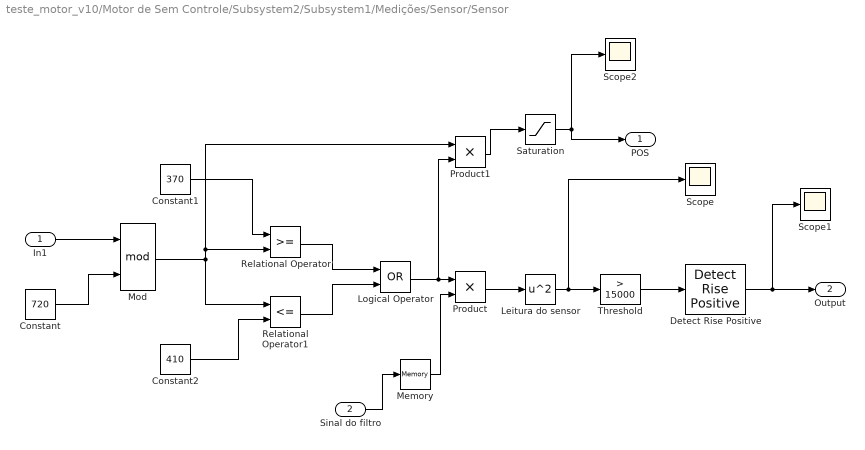
== system teste_motor_v10/Motor de Sem Controle/Subsystem2/Subsystem1/Medições/Sensor/Sensor ==
  In1 : Inport
  Sinal do filtro : Inport  Port=2
  Constant : Constant  Value=720
  Constant1 : Constant  Value=370
  Constant2 : Constant  Value=410
  Detect Rise Positive : simulink/Logic and Bit Operations/Detect Rise Positive  vinit=0  OutDataTypeStr=boolean
  Leitura do sensor : Math  Operator=square
  Logical Operator : Logic  Operator=OR  AllPortsSameDT=off  OutDataTypeStr=boolean
  Memory : Memory
  Mod : Math  Operator=mod
  Product : Product
  Product1 : Product
  Relational Operator : RelationalOperator  OutDataTypeStr=boolean  RndMeth=Simplest  InputSameDT=off
  Relational Operator1 : RelationalOperator  Operator=<=  OutDataTypeStr=boolean  RndMeth=Simplest  InputSameDT=off
  Saturation : Saturate  UpperLimit=450  LowerLimit=300
  Scope : Scope
      settings: ActiveDisplayYMinimum=14367.56981  ActiveDisplayYMaximum=16565.8865
  Scope1 : Scope
      settings: ActiveDisplayYMinimum=-0.125  ActiveDisplayYMaximum=1.125  DataLoggingVariableName=ScopeData6
  Scope2 : Scope
      settings: ActiveDisplayYMinimum=286.25  ActiveDisplayYMaximum=423.75
  Threshold : simulink/Logic and Bit Operations/Compare To Constant  relop=>  const=15000  OutDataTypeStr=boolean
  POS : Outport
  Output : Outport  Port=2
  wires:
  Relational Operator1/1 -> Logical Operator/2
  Relational Operator/1 -> Logical Operator/1
  Constant1/1 -> Relational Operator/1
  Mod/1 -> Product1/1, Relational Operator/2, Relational Operator1/1
  Constant2/1 -> Relational Operator1/2
  Detect Rise Positive/1 -> Scope1/1, Output/1
  Constant/1 -> Mod/2
  Leitura do sensor/1 -> Scope/1, Threshold/1
  Product/1 -> Leitura do sensor/1
  Threshold/1 -> Detect Rise Positive/1
  In1/1 -> Mod/1
  Sinal do filtro/1 -> Memory/1
  Memory/1 -> Product/2
  Logical Operator/1 -> Product1/2, Product/1
  Product1/1 -> Saturation/1
  Saturation/1 -> Scope2/1, POS/1

== system teste_motor_v10/Motor de Sem Controle/Subsystem2/Subsystem1/Medições/Sensor/Subsystem4 ==
  u : Inport
  Scope : Scope
      settings: ActiveDisplayYMinimum=-1310.25  ActiveDisplayYMaximum=11792.25  DataLoggingVariableName=ScopeData4
  Subsystem : Subsystem
  Subsystem1 : Subsystem
  Subsystem3 : Subsystem
  Out1 : Outport
  wires:
  u/1 -> Subsystem3/1(In1), Subsystem1/1(u), Subsystem/1(u)
  Subsystem1/1(Contagem) -> Scope/1, Subsystem3/2(u)
  Subsystem3/1(Out1) -> Out1/1
  Subsystem/1(Borda de Subida) -> Subsystem3/3(In3)

== system teste_motor_v10/Motor de Sem Controle/Subsystem2/Subsystem1/Medições/Filtro/Subsystem1/Subsystem ==
  Rel Spark : Inport
  RPM : Inport  Port=2
  2-D Lookup Table : Lookup_n-D  BreakpointsForDimension1=[12, 17, 20, 25, 30]  BreakpointsForDimension2=[200, 400, 800, 1000, 2000]  Table=[0 0 0 0 0; 0.05 0.05 0.02 0.01 0.01; 0.2 0.15 0.1 0.05 0.05; 0.6 0.5 0.3 0.2 0.1; 0.95 0.9 0.8 0.6 0.4]  InternalRulePriority=Speed  RndMeth=Simplest
      settings: InputPortMap=u0,u1
  Constant4 : Constant
  Relational Operator : RelationalOperator  Operator=<  OutDataTypeStr=boolean  RndMeth=Simplest  InputSameDT=off
  Subtract : Sum  Inputs=+-
  Uniform Random Number : UniformRandomNumber  Minimum=0  SampleTime=0.1
  Unit Delay : UnitDelay  SampleTime=-1  HasFrameUpgradeWarning=on
  knock : Outport
  wires:
  2-D Lookup Table/1 -> Subtract/2
  RPM/1 -> 2-D Lookup Table/2
  Relational Operator/1 -> Unit Delay/1
  Unit Delay/1 -> knock/1
  Rel Spark/1 -> 2-D Lookup Table/1
  Uniform Random Number/1 -> Relational Operator/2
  Subtract/1 -> Relational Operator/1
  Constant4/1 -> Subtract/1
